simulink model "ex4"  (Simulink 6.3)
settings: Solver=ode45  StartTime=0.0  StopTime=10000  RelTol=1e-3
values from neighbouring files (symbols this model uses):
  SymbolRate = 1000    [ex11.m]    (also in ex2sim.m = 2; ex4sim.m = 2; ex7sim.m = 2)
libraries: dspbuff3 x4, commutil2 x4, commsink2 x2, commfilt2 x2, commdigbbndpm2 x2, commchan3 x1, commrandsrc2 x1
settings Model: LastModifiedBy=lxy  StrictBusMsg=None
settings OptimizationCC: InlineInvariantSignals=on

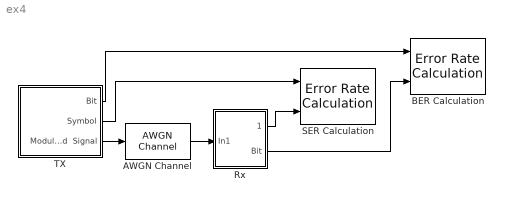
== system ex4 ==
  AWGN Channel : commchan3/AWGN Channel  seed=1111  noiseMode="Signal to noise ratio  (Es/No)"  EbNodB=10  EsNodB=SNR  SNRdB=10  bitsPerSym=1  Ps=1  Tsym=1/SymbolRate  variance=1
  BER Calculation : commsink2/Error Rate Calculation  N=0  st_delay=4*SymbolRate  cp_mode=Entire frame  subframe=[]  PMode=Workspace  WsName=BER  RsMode2=off  stop=off  numErr=100  maxBits=1e6
  Rx : Subsystem
  SER Calculation : commsink2/Error Rate Calculation  N=0  st_delay=SymbolRate  cp_mode=Entire frame  subframe=[]  PMode=Workspace  WsName=SER  RsMode2=off  stop=off  numErr=100  maxBits=1e6
  TX : Subsystem
  wires:
  TX/3(Modulated  Signal) -> AWGN Channel/1
  TX/2(Symbol) -> SER Calculation/1
  Rx/1(Symbol) -> SER Calculation/2
  Rx/2(Bit) -> BER Calculation/2
  TX/1(Bit) -> BER Calculation/1
  AWGN Channel/1 -> Rx/1(In1)

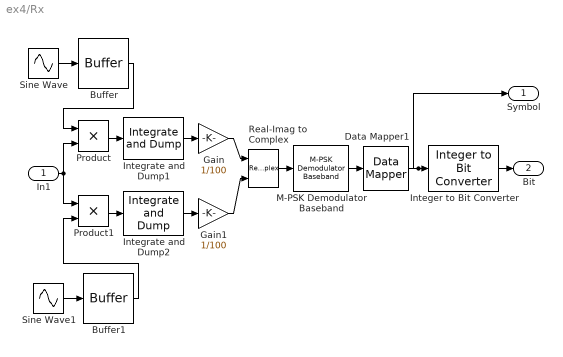
== system ex4/Rx ==
  In1 : Inport
  Buffer : dspbuff3/Buffer  N=100*SymbolRate  V=0  ic=0
  Buffer1 : dspbuff3/Buffer  N=100*SymbolRate  V=0  ic=0
  Data Mapper1 : commutil2/Data Mapper  MapMode=Gray to Binary  M=16  MapVec=[0 1 3 2 7 6 4 5]
  Gain : Gain  Gain=1/100
  Gain1 : Gain  Gain=1/100
  Integer to Bit Converter : commutil2/Integer to Bit Converter  nbits=4  outDtype=Same as input
  Integrate and Dump1 : commfilt2/Integrate and Dump  obssamples=100  offsetsamples=0  nodump=off
  Integrate and Dump2 : commfilt2/Integrate and Dump  obssamples=100  offsetsamples=0  nodump=off
  M-PSK Demodulator Baseband : commdigbbndpm2/M-PSK Demodulator Baseband  M=16  OutType=Integer  Dec=Binary  Ph=0  numSamp=1
  Product : Product  OutDataTypeMode=double  RndMeth=Zero
  Product1 : Product  OutDataTypeMode=double  RndMeth=Zero
  Real-Imag to Complex : RealImagToComplex
  Sine Wave : Sin  Amplitude=sqrt(2)  Frequency=2*pi*SymbolRate  Phase=pi/2  Samples=100  SampleTime=1/(100*SymbolRate)
  Sine Wave1 : Sin  Amplitude=sqrt(2)  Frequency=2*pi*SymbolRate  Phase=pi  Samples=100  SampleTime=1/(100*SymbolRate)
  Symbol : Outport
  Bit : Outport  Port=2
  wires:
  Integer to Bit Converter/1 -> Bit/1
  M-PSK Demodulator Baseband/1 -> Data Mapper1/1
  Real-Imag to Complex/1 -> M-PSK Demodulator Baseband/1
  Integrate and Dump1/1 -> Gain/1
  Gain/1 -> Real-Imag to Complex/1
  Product/1 -> Integrate and Dump1/1
  Sine Wave/1 -> Buffer/1
  Buffer/1 -> Product/1
  Sine Wave1/1 -> Buffer1/1
  Buffer1/1 -> Product1/2
  Integrate and Dump2/1 -> Gain1/1
  Gain1/1 -> Real-Imag to Complex/2
  Product1/1 -> Integrate and Dump2/1
  Data Mapper1/1 -> Symbol/1, Integer to Bit Converter/1
  In1/1 -> Product/2, Product1/1

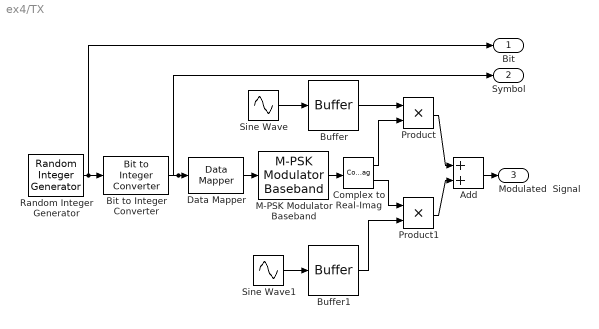
== system ex4/TX ==
  Add : Sum  OutScaling=2^-10
  Bit to Integer Converter : commutil2/Bit to Integer Converter  nbits=4  outDtype=Same as input
  Buffer : dspbuff3/Buffer  N=100*SymbolRate  V=0  ic=0
  Buffer1 : dspbuff3/Buffer  N=100*SymbolRate  V=0  ic=0
  Complex to Real-Imag : ComplexToRealImag
  Data Mapper : commutil2/Data Mapper  MapMode=Binary to Gray  M=16  MapVec=[0 1 3 2 7 6 4 5]
  M-PSK Modulator Baseband : commdigbbndpm2/M-PSK Modulator Baseband  M=16  InType=Integer  Enc=Binary  Ph=0  numSamp=100
  Product : Product  RndMeth=Zero
  Product1 : Product  RndMeth=Zero
  Random Integer Generator : commrandsrc2/Random Integer Generator  mul=2  seed=37  Ts=1/(4*SymbolRate)  frameBased=on  sampPerFrame=4*SymbolRate  orient=off  outDataType=double
  Sine Wave : Sin  Amplitude=sqrt(2)  Frequency=2*pi*SymbolRate  Phase=pi/2  Samples=100  SampleTime=1/(100*SymbolRate)
  Sine Wave1 : Sin  Amplitude=sqrt(2)  Frequency=2*pi*SymbolRate  Phase=pi  Samples=100  SampleTime=1/(100*SymbolRate)
  Bit : Outport
  Symbol : Outport  Port=2
  Modulated  Signal : Outport  Port=3
  wires:
  Data Mapper/1 -> M-PSK Modulator Baseband/1
  M-PSK Modulator Baseband/1 -> Complex to Real-Imag/1
  Complex to Real-Imag/1 -> Product/2
  Sine Wave/1 -> Buffer/1
  Buffer/1 -> Product/1
  Sine Wave1/1 -> Buffer1/1
  Buffer1/1 -> Product1/2
  Complex to Real-Imag/2 -> Product1/1
  Product/1 -> Add/1
  Product1/1 -> Add/2
  Add/1 -> Modulated  Signal/1
  Random Integer Generator/1 -> Bit to Integer Converter/1, Bit/1
  Bit to Integer Converter/1 -> Data Mapper/1, Symbol/1
